simulink model "flcClosedSystem"  (R2021a)
settings: Solver=VariableStepAuto  StartTime=0.0  StopTime=20.0  RelTol=1e-3
libraries: SignalEditorBlockLib x1, checkpacklib x1
settings Model: Creator=vash  LastModifiedBy=vash

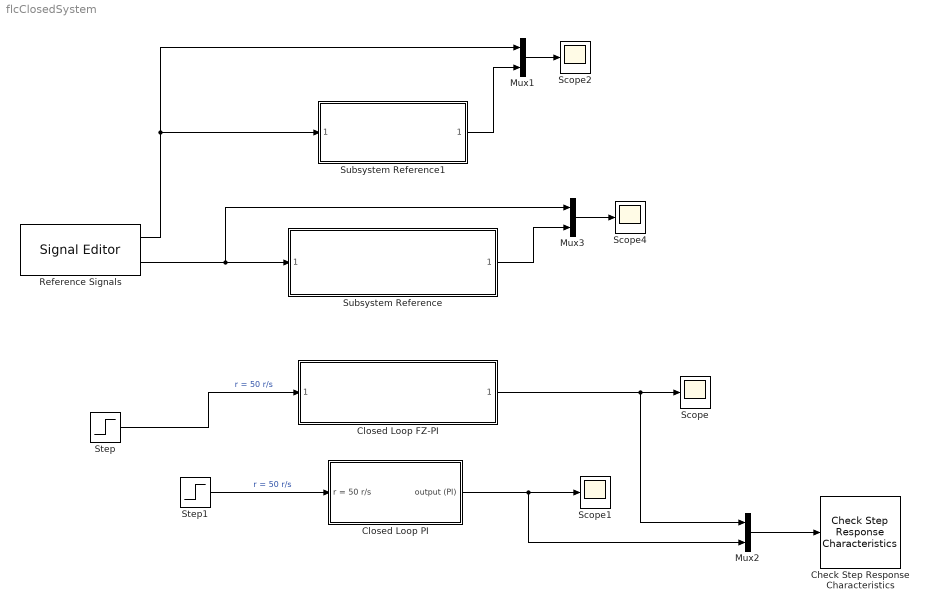
== system flcClosedSystem ==
  " Reference Signals" : SignalEditorBlockLib/Signal Editor  FileName=customReferenceSignals.mat  ActiveScenario=Scenario  ActiveSignal=Trapezoid  IsBus=off  OutputBusObjectStr=Bus: BusObject  SampleTime=0  ZeroCross=off  OutputAfterFinalValue=Setting to zero  Unit=inherit  PreserveSignalName=on
  Check Step Response Characteristics : checkpacklib/Check Step Response  Characteristics  InstantiateOnLoad=on  enabled=on  stopWhenAssertionFail=off  export=off  ViewDlgPos=[1921 31 1920 973]  OpenViewOnLoad=off  LaunchViewOnOpen=off  TimeUnits=seconds  EnableStepResponseBound=on  InitialValue=0  FinalValue=50  StepTime=0  RiseTime=0.6  PercentRise=80  SettlingTime=9  PercentSettling=3  PercentOvershoot=6  PercentUndershoot=1
      settings: SourceProductBaseCode=CT,ID,MT,SO
  Closed Loop FZ-PI : Subsystem  ReferencedSubsystem=Closed_Loop_FZ_PI
  Closed Loop PI : Subsystem
  Mux1 : Mux  Inputs=2
  Mux2 : Mux  Inputs=2
  Mux3 : Mux  Inputs=2
  Scope{,1..2,4} (4 alike) : Scope
  Step : Step  Before=50  After=50  SampleTime=0
  Step1 : Step  Before=50  After=50  SampleTime=0
  Subsystem Reference : Subsystem  ReferencedSubsystem=Closed_Loop_FZ_PI
  Subsystem Reference1 : Subsystem  ReferencedSubsystem=Closed_Loop_FZ_PI
  wires:
  Mux2/1 -> Check Step Response Characteristics/1
  Closed Loop FZ-PI/1 -> Mux2/1, Scope/1
  Closed Loop PI/1(output (PI)) -> Scope1/1, Mux2/2
  Step1/1 -> Closed Loop PI/1(r = 50 r/s)  "r = 50 r/s"
  " Reference Signals"/1 -> Mux1/1, Subsystem Reference1/1
  " Reference Signals"/2 -> Mux3/1, Subsystem Reference/1
  Step/1 -> Closed Loop FZ-PI/1  "r = 50 r/s"
  Mux1/1 -> Scope2/1
  Subsystem Reference1/1 -> Mux1/2
  Mux3/1 -> Scope4/1
  Subsystem Reference/1 -> Mux3/2

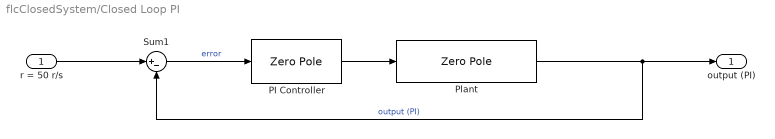
== system flcClosedSystem/Closed Loop PI ==
  r = 50 r/s : Inport
  PI Controller : ZeroPole  Zeros=[-0.35]  Poles=[0]  Gain=1
  Plant : ZeroPole  Zeros=[]  Poles=[-0.1 -10]  Gain=25
  Sum1 : Sum  Inputs=|+-
  output (PI) : Outport
  wires:
  PI Controller/1 -> Plant/1
  Plant/1 -> Sum1/2, output (PI)/1  "output (PI)"
  r = 50 r/s/1 -> Sum1/1
  Sum1/1 -> PI Controller/1  "error"
